simulink model "Q3_Impulse"  (R2026a)
settings: Solver=ode45  StopTime=2  RelTol=1e-8  AbsTol=1e-10
model workspace (MAT data in the model file):
  input_signal = timeseries
  input_signal.Name = 'unnamed'
  input_signal.DataInfo = tsdata.datametadata
  input_signal.DataInfo.Interpolation = tsdata.interpolation
  input_signal.DataInfo.Interpolation.Fhandle : function handle (value not decoded)
  input_signal.DataInfo.Interpolation.Name = 'linear'
  input_signal.TimeInfo = tsdata.timemetadata
  input_signal.TimeInfo.Length = 4001
  input_signal.TimeInfo.DuplicateTimes = 0
  input_signal.TimeInfo.Time_ = [0 0.0005 0.001 0.0015 0.002 0.0025 0.003 0.0035 0.004 0.0045 0.005 0.0055 ... (4001 elements, 4001x1)]
  input_signal.TimeInfo.Initialized = 1
  input_signal.QualityInfo = tsdata.qualmetadata
  input_signal.Data_ = [500 500 500 500 0 0 0 0 0 0 0 0 ... (4001 elements, 4001x1)]
settings Model: Creator=szj  LastModifiedBy=szj

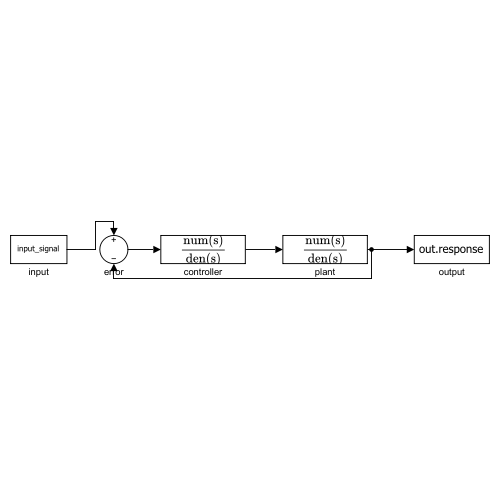
[thumbnail: Simulink's stored preview of the top-level diagram]
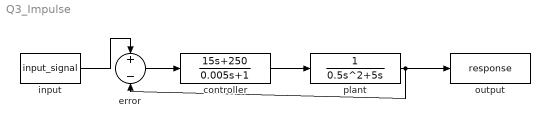
== system Q3_Impulse ==
  controller : TransferFcn  Numerator=[15 250]  Denominator=[0.005 1]
  error : Sum  Inputs=+-
  input : FromWorkspace  VariableName=input_signal
  output : ToWorkspace  VariableName=response  SaveFormat=Timeseries  SampleTime=-1
  plant : TransferFcn  Numerator=[0 0 1]  Denominator=[0.5 5 0]
  wires:
  input/1 -> error/1
  error/1 -> controller/1
  controller/1 -> plant/1
  plant/1 -> output/1, error/2
